simulink library "Propulsion_Lib"  (Simulink 7.5)
settings: Solver=ode45  SolverMode=SingleTasking  StartTime=0.0  StopTime=10.0  RelTol=1e-3
values from neighbouring files (symbols this model uses):
  AC = FASER_config    [UAV_config.m]    (also in UAV_modelconfig.mat = )
  TrimCondition =     [UAV_trimcondition.mat]
libraries: simulink x2, aerolibutil x1, aerolibbdyn x1, aerolibtransform2 x1
settings Model: Creator=Paul Freeman  LastModifiedBy=austinmurch

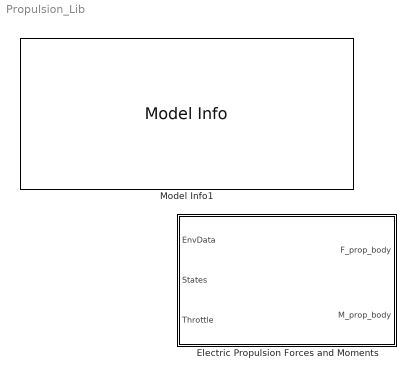
== system Propulsion_Lib ==
  Electric Propulsion Forces and Moments : Subsystem
  Model Info1 : simulink/Model-Wide Utilities/Model Info  SystemSampleTime=-1  InitialBlockCM=None  BlockCM=None  Frame=on  DisplayStringWithTags=|  HorizontalTextAlignment=Left  LeftAlignmentValue=0.02  SourceBlockDiagram=Propulsion_Lib  TagMaxNumber=20
      | MODEL INFORMATION
      | Propulsion Library
      | 
      | University of Minnesota
      | Aerospace Engineering and Mechanics
      | Copyright 2011 Regents of the University of Minnesota. All rights reserved.
      | 
      | == SVN Info ==
      | %<ModelVersion>
      | Last modified by %<LastModifiedBy> on %<LastModificationDate>

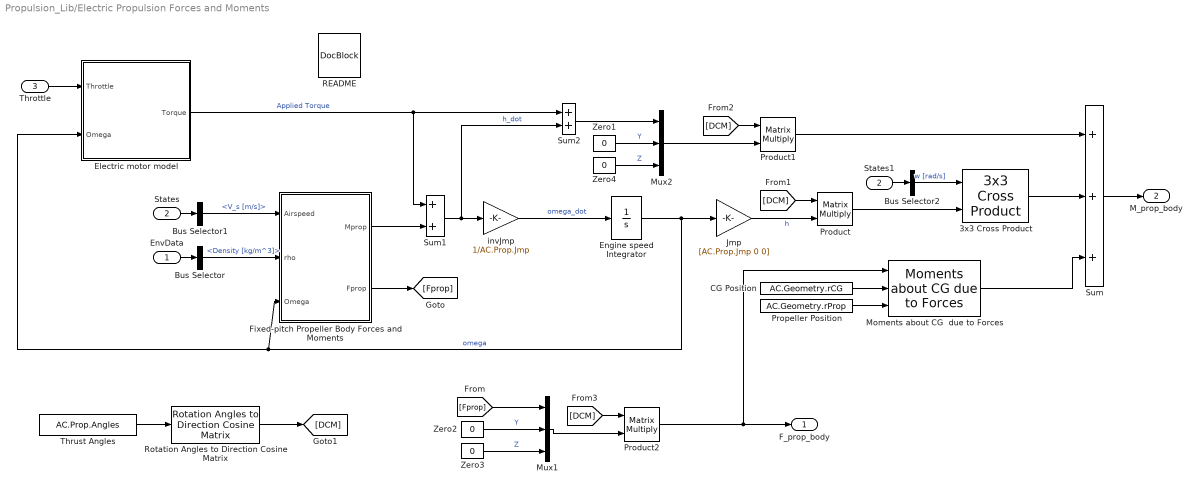
== system Propulsion_Lib/Electric Propulsion Forces and Moments ==
  EnvData : Inport  OutDataType=sfix(16)  OutScaling=2^0
  States : Inport  Port=2  OutDataType=sfix(16)  OutScaling=2^0
  Throttle : Inport  Port=3  DataType=double  OutDataType=sfix(16)  OutScaling=2^0  OutDataTypeStr=double
  3x3 Cross Product : aerolibutil/3x3 Cross Product  SystemSampleTime=-1
  Bus Selector : BusSelector  OutputSignals=Density [kg/m^3]
  Bus Selector1 : BusSelector  OutputSignals=WindAxesParam.V_s [m/s]
  Bus Selector2 : BusSelector  OutputSignals=AngVel [rad/s].p [rad/s],AngVel [rad/s].q [rad/s],AngVel [rad/s].r [rad/s]  OutputAsBus=on
  CG Position : Constant  Value=AC.Geometry.rCG  OutDataType=sfix(16)  OutScaling=2^0
  Electric motor model : Subsystem
  Engine speed Integrator : Integrator  InitialCondition=TrimCondition.EngineSpeedIni  LimitOutput=on  UpperSaturationLimit=AC.Prop.OmegaSaturation.Upper  LowerSaturationLimit=AC.Prop.OmegaSaturation.Lower
  Fixed-pitch Propeller Body Forces and Moments : Subsystem
  Jmp : Gain  Gain=[AC.Prop.Jmp 0 0]  ParameterDataType=sfix(16)  ParameterScaling=2^0  OutDataType=sfix(16)  OutScaling=2^0  SaturateOnIntegerOverflow=on  OutDataTypeStr=Inherit: Same as input  ParamDataTypeStr=Inherit: Same as input
  Moments about CG  due to Forces : aerolibbdyn/Moments about CG  due to Forces  SystemSampleTime=-1
  Mux1 : Mux  Inputs=3
  Mux2 : Mux  Inputs=3
  Product : Product  Multiplication=Matrix(*)  OutDataType=fixdt(1, 16)  OutScaling=2^0  RndMeth=Zero
  Product1 : Product  Multiplication=Matrix(*)  OutDataType=fixdt(1, 16)  OutScaling=2^0  RndMeth=Zero
  Product2 : Product  Multiplication=Matrix(*)  OutDataType=fixdt(1, 16)  OutScaling=2^0  RndMeth=Zero
  Propeller Position : Constant  Value=AC.Geometry.rProp  OutDataType=sfix(16)  OutScaling=2^0
  README : simulink/Model-Wide Utilities/DocBlock  SystemSampleTime=-1  DocumentType=Text
      content=|
      | Electric Propulsion Forces and Moments
      |
      | This block models the electric motor, propeller, and the resulting forces
      | and moments.
      |
      | The electric motor is modeled by using a table lookup to relate throttle
      | position to power output in Watts; power is coverted to torque by
      | dividing by the current motor angular velocity, omega (rad/s). This
      | torque is then summed with the required torque from the propeller. The
      | resulting net torque is divided by the combined motor/propeller inertia,
      | yielding omega_dot, which is integrated to get the current motor speed.
      | The initial condition of the Engine speed integrator is set in the
      | TrimCondition data structure.
      |
      | The propeller is modelled using lookup tables of Thrust and Power
      | Coefficients, CT and CP, as a function of advance ratio J. These are
      | defined as:
      |
      | CT = Thrust / (R^4 * omega^2 * 4/pi^2 * rho)
      | CP = Power  / (R^5 * omega^3 * 4/pi^3 * rho)
      | J  = V * pi / (omega * R)
      |
      | where R is the propeller radius, omega is the angular velocity in
      | radians per second, and rho is the density of air. Note that the
      | torque coefficient for the propeller can be calculated from CP by
      | multiplying by n; thus the torque coefficient is not explicitly modeled.
      |
      | The total forces due to the propeller is simply the thrust, which is
      | not directly aligned with the body axes, so it must be rotated. These
      | angles are set in the aircraft configuration m-file.
      |
      | The moments due to the propeller are due to the derivative of the angular
      | momemtum (ie gyroscopic moments) and moments due to the position of the
      | thrustline relative to the center of gravity. In addition, the torque from
      | the motor appears as an applied moment in the equations of motion. The
      | moments due to the propeller are as follows:
      |
      | Mp = d/dt(Jmp*omega) + M_motor
      |
      | where Jmp is the moment of inertia of the rotating portion of the motor
      | and propeller. Taking the derivative in the body frame, which is
      | non-inertial, results in:
      |
      | Mp = Jmp*omega_dot + [p;q;r] X omega*Jmp + M_motor
      |
      | where [p;q;r] is the body axis angular velocity. Since the
      | rotation axis is NOT aligned with the body x-axis, we must rotate these the
      | angular moment terms by a rotation matrix (L_mb) before computing the cross
      | product:
      |
      | Mp = L_mb*(Jmp*omega_dot + M_motor) + [p;q;r] X L_mb*omega*Jmp
      |
      | The data for the lookup tables and all of the needed aircraft parameters
      | are stored in the aircraft configuration data structure (AC).
      |
      | >> AC.Prop
      |
      | ans =
      |
      |                      CT: [-0.4314 1.0800 -0.8960 0.1089 0.0604]
      |                      CP: [0.5054 -0.5304 0.0412 0.0166 0.0223]
      |                  Radius: 0.1524
      |                   Power: [174.4600 70.1350 -4.3900]
      |     ThrottleOutputLimit: [1x1 struct]
      |         OmegaSaturation: [1x1 struct]
      |                     Jmp: 1.2991e-004
      |                  Angles: [0 0 0.0524]
  Rotation Angles to Direction Cosine Matrix : aerolibtransform2/Rotation Angles to Direction Cosine Matrix  SystemSampleTime=-1  rotationOrder=ZYX
  States1 : InportShadow  Port=2  OutDataType=sfix(16)  OutScaling=2^0
  Sum : Sum  Inputs=+++  OutDataType=sfix(16)  OutScaling=2^0
  Sum1 : Sum  OutDataType=sfix(16)  OutScaling=2^0  SaturateOnIntegerOverflow=on  InputSameDT=on  OutDataTypeStr=Inherit: Same as first input
  Sum2 : Sum  OutDataType=sfix(16)  OutScaling=2^0
  Thrust Angles : Constant  Value=AC.Prop.Angles  OutDataType=sfix(16)  OutScaling=2^0
  Zero{1..4} (4 alike) : Constant  Value=0  OutDataType=sfix(16)  OutScaling=2^0
  invJmp : Gain  Gain=1/AC.Prop.Jmp  ParameterDataType=sfix(16)  ParameterScaling=2^0  OutDataType=sfix(16)  OutScaling=2^0
  F_prop_body : Outport  OutDataType=sfix(16)  OutScaling=2^0
  M_prop_body : Outport  Port=2  OutDataType=sfix(16)  OutScaling=2^0
  wires:
  invJmp/1 -> Engine speed Integrator/1  "omega_dot"
  Sum1/1 -> invJmp/1, Sum2/2  "h_dot"
  Throttle/1 -> Electric motor model/1(Throttle)
  Electric motor model/1(Torque) -> Sum1/1, Sum2/1  "Applied Torque"
  Engine speed Integrator/1 -> Electric motor model/2(Omega), Fixed-pitch Propeller Body Forces and Moments/3(Omega), Jmp/1  "omega"
  Zero3/1 -> Mux1/3  "Z"
  Zero2/1 -> Mux1/2  "Y"
  EnvData/1 -> Bus Selector/1
  States/1 -> Bus Selector1/1
  CG Position/1 -> Moments about CG  due to Forces/2
  Propeller Position/1 -> Moments about CG  due to Forces/3
  Sum/1 -> M_prop_body/1
  States1/1 -> Bus Selector2/1
  [Fprop] -> Mux1/1
  Bus Selector1/1 -> Fixed-pitch Propeller Body Forces and Moments/1(Airspeed)  "<V_s [m/s]>"
  Bus Selector/1 -> Fixed-pitch Propeller Body Forces and Moments/2(rho)  "<Density [kg/m^3]>"
  Fixed-pitch Propeller Body Forces and Moments/1(Mprop) -> Sum1/2
  Fixed-pitch Propeller Body Forces and Moments/2(Fprop) -> [Fprop]
  Jmp/1 -> Product/2  "h"
  Bus Selector2/1 -> 3x3 Cross Product/1  "w [rad/s]"
  Thrust Angles/1 -> Rotation Angles to Direction Cosine Matrix/1
  Rotation Angles to Direction Cosine Matrix/1 -> [DCM]
  [DCM] -> Product/1
  [DCM] -> Product1/1
  [DCM] -> Product2/1
  Mux1/1 -> Product2/2
  Product2/1 -> Moments about CG  due to Forces/1, F_prop_body/1
  Product/1 -> 3x3 Cross Product/2
  Zero4/1 -> Mux2/3  "Z"
  Zero1/1 -> Mux2/2  "Y"
  Sum2/1 -> Mux2/1
  Mux2/1 -> Product1/2
  Product1/1 -> Sum/1
  3x3 Cross Product/1 -> Sum/2
  Moments about CG  due to Forces/1 -> Sum/3

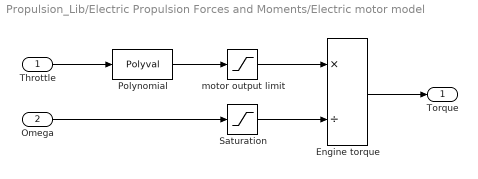
== system Propulsion_Lib/Electric Propulsion Forces and Moments/Electric motor model ==
  Throttle : Inport  DataType=double  OutDataType=sfix(16)  OutScaling=2^0  OutDataTypeStr=double
  Omega : Inport  Port=2  DataType=double  OutDataType=sfix(16)  OutScaling=2^0  OutDataTypeStr=double
  Engine torque : Product  Inputs=*/  OutDataType=sfix(16)  OutScaling=2^0  SaturateOnIntegerOverflow=on  InputSameDT=on  OutDataTypeStr=Inherit: Same as first input
  Polynomial : Polyval  Coefs=AC.Prop.Power
  Saturation : Saturate  UpperLimit=AC.Prop.OmegaSaturation.Upper  LowerLimit=AC.Prop.OmegaSaturation.Lower
  motor output limit : Saturate  UpperLimit=AC.Prop.ThrottleOutputLimit.Upper  LowerLimit=AC.Prop.ThrottleOutputLimit.Lower
  Torque : Outport  OutDataType=sfix(16)  OutScaling=2^0
  wires:
  Saturation/1 -> Engine torque/2
  Engine torque/1 -> Torque/1
  Omega/1 -> Saturation/1
  Polynomial/1 -> motor output limit/1
  Throttle/1 -> Polynomial/1
  motor output limit/1 -> Engine torque/1

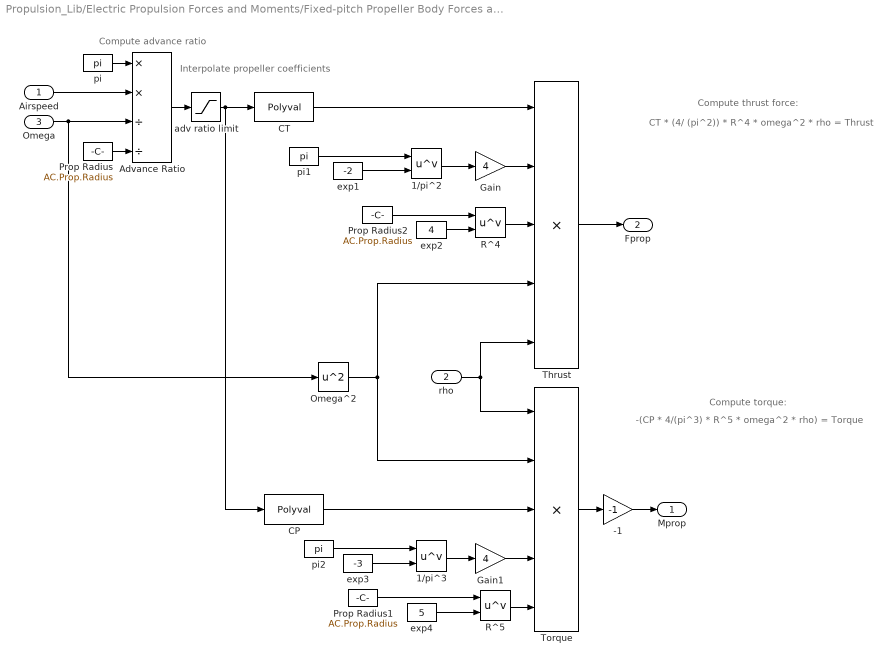
== system Propulsion_Lib/Electric Propulsion Forces and Moments/Fixed-pitch Propeller Body Forces and Moments ==
  note: Compute torque:
  note: Interpolate propeller coefficients
  note: Compute thrust force:
  note: Compute advance ratio
  note: CT * (4/ (pi^2)) * R^4 * omega^2 * rho = Thrust
  note: -(CP * 4/(pi^3) * R^5 * omega^2 * rho) = Torque
  Airspeed : Inport  DataType=double  OutDataType=sfix(16)  OutScaling=2^0  OutDataTypeStr=double
  rho : Inport  Port=2  DataType=double  OutDataType=sfix(16)  OutScaling=2^0  OutDataTypeStr=double
  Omega : Inport  Port=3  DataType=double  OutDataType=sfix(16)  OutScaling=2^0  OutDataTypeStr=double
  -1 : Gain  Gain=-1  ParameterDataType=sfix(16)  ParameterScaling=2^0  OutDataType=sfix(16)  OutScaling=2^0  SaturateOnIntegerOverflow=on  OutDataTypeStr=Inherit: Same as input  ParamDataTypeStr=Inherit: Same as input
  1/pi^2 : Math  Operator=pow  OutDataType=sfix(16)  OutScaling=2^0  SaturateOnIntegerOverflow=on
  1/pi^3 : Math  Operator=pow  OutDataType=sfix(16)  OutScaling=2^0  SaturateOnIntegerOverflow=on
  Advance Ratio : Product  Inputs=**//  OutDataType=sfix(16)  OutScaling=2^0  SaturateOnIntegerOverflow=on  InputSameDT=on  OutDataTypeStr=Inherit: Same as first input
  CP : Polyval  Coefs=AC.Prop.CP
  CT : Polyval  Coefs=AC.Prop.CT
  Gain : Gain  Gain=4  ParameterDataType=sfix(16)  ParameterScaling=2^0  OutDataType=sfix(16)  OutScaling=2^0  SaturateOnIntegerOverflow=on  OutDataTypeStr=Inherit: Same as input  ParamDataTypeStr=Inherit: Same as input
  Gain1 : Gain  Gain=4  ParameterDataType=sfix(16)  ParameterScaling=2^0  OutDataType=sfix(16)  OutScaling=2^0  SaturateOnIntegerOverflow=on  OutDataTypeStr=Inherit: Same as input  ParamDataTypeStr=Inherit: Same as input
  Omega^2 : Math  Operator=square  OutDataType=sfix(16)  OutScaling=2^0  SaturateOnIntegerOverflow=on
  Prop Radius : Constant  Value=AC.Prop.Radius  OutDataType=sfix(16)  OutScaling=2^0
  Prop Radius1 : Constant  Value=AC.Prop.Radius  OutDataType=sfix(16)  OutScaling=2^0
  Prop Radius2 : Constant  Value=AC.Prop.Radius  OutDataType=sfix(16)  OutScaling=2^0
  R^4 : Math  Operator=pow  OutDataType=sfix(16)  OutScaling=2^0  SaturateOnIntegerOverflow=on
  R^5 : Math  Operator=pow  OutDataType=sfix(16)  OutScaling=2^0  SaturateOnIntegerOverflow=on
  Thrust : Product  Inputs=5  OutDataType=sfix(16)  OutScaling=2^0  SaturateOnIntegerOverflow=on  InputSameDT=on  OutDataTypeStr=Inherit: Same as first input
  Torque : Product  Inputs=5  OutDataType=sfix(16)  OutScaling=2^0  SaturateOnIntegerOverflow=on  InputSameDT=on  OutDataTypeStr=Inherit: Same as first input
  adv ratio limit : Saturate  UpperLimit=0.7  LowerLimit=0
  exp1 : Constant  Value=-2  OutDataType=sfix(16)  OutScaling=2^0
  exp2 : Constant  Value=4  OutDataType=sfix(16)  OutScaling=2^0
  exp3 : Constant  Value=-3  OutDataType=sfix(16)  OutScaling=2^0
  exp4 : Constant  Value=5  OutDataType=sfix(16)  OutScaling=2^0
  pi : Constant  Value=pi  OutDataType=sfix(16)  OutScaling=2^0
  pi1 : Constant  Value=pi  OutDataType=sfix(16)  OutScaling=2^0
  pi2 : Constant  Value=pi  OutDataType=sfix(16)  OutScaling=2^0
  Mprop : Outport  OutDataType=sfix(16)  OutScaling=2^0
  Fprop : Outport  Port=2  OutDataType=sfix(16)  OutScaling=2^0
  wires:
  CP/1 -> Torque/3
  CT/1 -> Thrust/1
  Torque/1 -> -1/1
  Thrust/1 -> Fprop/1
  Gain1/1 -> Torque/4
  Gain/1 -> Thrust/2
  R^5/1 -> Torque/5
  exp4/1 -> R^5/2
  R^4/1 -> Thrust/3
  exp2/1 -> R^4/2
  1/pi^3/1 -> Gain1/1
  1/pi^2/1 -> Gain/1
  exp3/1 -> 1/pi^3/2
  Omega^2/1 -> Thrust/4, Torque/2
  Advance Ratio/1 -> adv ratio limit/1
  Prop Radius/1 -> Advance Ratio/4
  pi1/1 -> 1/pi^2/1
  Omega/1 -> Omega^2/1, Advance Ratio/3
  rho/1 -> Thrust/5, Torque/1
  Airspeed/1 -> Advance Ratio/2
  exp1/1 -> 1/pi^2/2
  Prop Radius1/1 -> R^5/1
  Prop Radius2/1 -> R^4/1
  pi2/1 -> 1/pi^3/1
  pi/1 -> Advance Ratio/1
  -1/1 -> Mprop/1
  adv ratio limit/1 -> CT/1, CP/1
